simulink model "Plant_sim"  (R2022b)
settings: Solver=VariableStepAuto  StartTime=0.0  StopTime=10.0  RelTol=1e-3
PreLoadFcn:
  | param
values from neighbouring files (symbols this model uses):
  b = 0.1    [init_cond.m]    (also in param.m)
  Ce = 1.2    [init_cond.m]    (also in param.m)
  Cm = 1.2    [init_cond.m]    (also in param.m)
  J = 0.04    [init_cond.m]    (also in param.m)
  Le = 0.01    [init_cond.m]    (also in param.m)
  Lf = 0.01    [init_cond.m]    (also in param.m)
  Lrot = Le+Lf    (= 0.02)    [init_cond.m]    (also in param.m)
  Re = 4    [init_cond.m]    (also in param.m)
  Rf = 0.9    [init_cond.m]    (also in param.m)
  Rrot = Re+Rf    (= 4.9)    [init_cond.m]    (also in param.m)
libraries: fl_lib x5, nesl_utility x4, ee_lib x1
settings Model: Creator=antsupove  LastModifiedBy=antsupove
settings DebuggingCC: UnconnectedInputMsg=warning  UnconnectedOutputMsg=warning  UnconnectedLineMsg=warning
settings ModelReferenceCC: EnableRefExpFcnMdlSchedulingChecks=on
settings RTWCC: DLArmComputeVersion=19.05

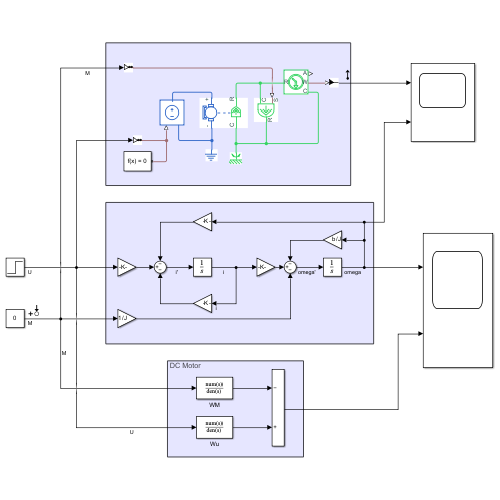
[thumbnail: Simulink's stored preview of the top-level diagram]
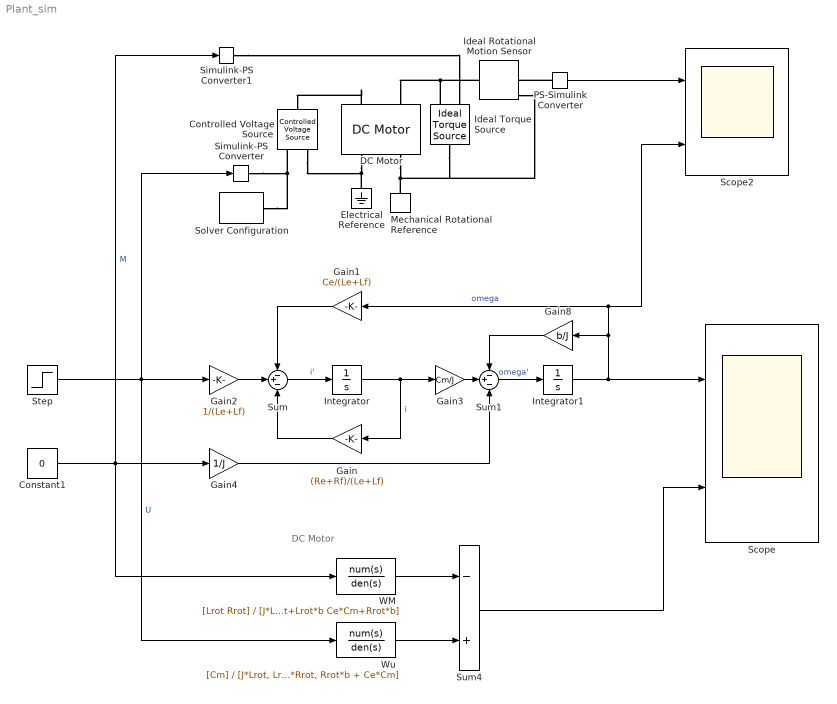
== system Plant_sim ==
  note: DC Motor
  Constant1 : Constant  Value=0
  Controlled Voltage Source : fl_lib/Electrical/Electrical Sources/Controlled Voltage Source
  DC Motor : ee_lib/Electromechanical/Brushed Motors/DC Motor  field_option=ee.enum.field_option.pm  Rf=100 Ohm  Lf=1 H  Laf=0.15 H  If0=0 A  parameterization=ee.enum.dcparam_option.circuit_param  Ra=Rrot Ohm  La=Lrot H  emf_or_torque=ee.enum.emf_or_torque.ki  Kv=0.072e-3 V/rpm  Ki=Cm N*m/A  T_stall=0.24e-3 N*m  w_max=19100 rpm  w_rated=15000 rpm  P_rated=0.08 W  V_rated=1.5 V  lam_param=ee.enum.lam_param.damping  i_noload=0 A  V_i_noload=1.5 V  J=J kg*m^2  lam=b N*m/(rad/s)  speed0=0 rad/s  enable_fault_armature=simscape.enum.onoff.off  rev_faulted=1 / 3  G_faulted_armature=1e-5 S  fault_trigger_armature=ee.enum.faults.faultTrigger.temporal  t_fault_armature=1 s  max_permissible_current_armature=inf A  t_fail_on_current_armature=1 s  enable_fault_field=simscape.enum.onoff.off  G_faulted_field=1e-5 S  fault_trigger_field=ee.enum.faults.faultTrigger.temporal  t_fault_field=1 s  max_permissible_current_field=inf A  t_fail_on_current_field=1 s  fault_action=simscape.enum.assert.action.none  alpha=3.93e-3 1/K  Tmeas=25 degC  thermal_mass=100 J/K  initial_temperature=25 degC
  Electrical Reference : fl_lib/Electrical/Electrical Elements/Electrical Reference
  Gain : Gain  Gain=(Re+Rf)/(Le+Lf)
  Gain1 : Gain  Gain=Ce/(Le+Lf)
  Gain2 : Gain  Gain=1/(Le+Lf)
  Gain3 : Gain  Gain=Cm/J
  Gain4 : Gain  Gain=1/J
  Gain8 : Gain  Gain=b/J
  Ideal Rotational Motion Sensor : fl_lib/Mechanical/Mechanical Sensors/Ideal Rotational Motion Sensor  reference=foundation.enum.MeasurementReference.difference  acceleration_port=false  velocity_port=true  position_port=true  wrap_angle=simscape.enum.onoff.off  offset=0 rad
  Ideal Torque Source : fl_lib/Mechanical/Mechanical Sources/Ideal Torque Source
  Integrator : Integrator
  Integrator1 : Integrator
  Mechanical Rotational Reference : fl_lib/Mechanical/Rotational Elements/Mechanical Rotational Reference
  PS-Simulink Converter : nesl_utility/PS-Simulink Converter  PhysicalDomain=network_engine_domain  SubClassName=ps_output  LeftPortType=input  RightPortType=output  PseudoPeriodic=off  Frequencies=[]  VectorFormat=1-D array  Unit=inherit  AffineConversion=off
  Scope : Scope  NumInputPorts=2
  Scope2 : Scope  NumInputPorts=2
  Simulink-PS Converter : nesl_utility/Simulink-PS Converter  PhysicalDomain=network_engine_domain  SubClassName=ps_input  LeftPortType=input  RightPortType=output  PseudoPeriodic=off  Frequencies=[]  NoiseDistribution=none  NoiseParameters=[]  Unit=1  AffineConversion=off  FilteringAndDerivatives=filter  SimscapeFilterOrder=2  InputFilterTimeConstant=0.001  UdotUserProvided=0
  Simulink-PS Converter1 : nesl_utility/Simulink-PS Converter  PhysicalDomain=network_engine_domain  SubClassName=ps_input  LeftPortType=input  RightPortType=output  PseudoPeriodic=off  Frequencies=[]  NoiseDistribution=none  NoiseParameters=[]  Unit=1  AffineConversion=off  FilteringAndDerivatives=filter  SimscapeFilterOrder=2  InputFilterTimeConstant=0.001  UdotUserProvided=0
  Solver Configuration : nesl_utility/Solver Configuration  PhysicalDomain=network_engine_domain  SubClassName=solver  LeftPortType=input  RightPortType=generic  Tones=[]  Harmonics=[]  SimulateNoise=off  Profile=off  UseLocalSampling=off  EnableSwitchedLinearOptims=on  FrequencyDomain=off  UseCCode=off  RelTol=0.001  AbsTol=1e-06  MinStep=1e-09  ToWorkspace=off  RevertToSquareIcSolve=off  NumHomotopyIterations=100  PhasorMode=off  PhasorModeNumHarmonics=1  ConsistencySolver=NEWTON_FTOL  IndexReductionMethod=DerivativeReplacement  DoDC=off  ResidualTolerance=1e-09  ConsistencyTolSource=GLOBAL  ConsistencyAbsTol=0.001  ConsistencyRelTol=0.001  ConsistencyTolFactor=0.001  UseLocalSolver=off  LocalSolverChoice=NE_BACKWARD_EULER_ADVANCER  ResolveIndetEquations=on  FunctionEvalNumThread=1  LocalSolverSampleTime=0.001  DoFixedCost=off  MaxNonlinIter=3  MaxModeIter=2  ComputeImpulses=off  ImpulseIterations=2  LinearAlgebra=auto  LinearAlgebraNumThread=0  EquationFormulation=NE_TIME_EF  DelaysMemoryBudget=1024  AutomaticFiltering=on  FilteringTimeConstant=0.001  PartitionStorageMethod=AS_NEEDED  PartitionMemoryBudget=1024  PartitionMethod=ROBUST
  Step : Step  SampleTime=0
  Sum : Sum  Inputs=-+-
  Sum1 : Sum  Inputs=-+-
  Sum4 : Sum  Inputs=-+
  WM : TransferFcn  Numerator=[Lrot Rrot]  Denominator=[J*Lrot J*Rrot+Lrot*b Ce*Cm+Rrot*b]
  Wu : TransferFcn  Numerator=[Cm]  Denominator=[J*Lrot, Lrot*b + J*Rrot, Rrot*b + Ce*Cm]
  wires:
  Sum/1 -> Integrator/1  "i'"
  Integrator/1 -> Gain/1, Gain3/1  "i"
  Integrator1/1 -> Scope2/2, Gain1/1, Gain8/1, Scope/1  "omega"
  Gain/1 -> Sum/3
  Gain1/1 -> Sum/1
  Gain2/1 -> Sum/2
  Sum1/1 -> Integrator1/1  "omega'"
  Step/1 -> Simulink-PS Converter/1, Gain2/1, Wu/1  "U"
  Sum4/1 -> Scope/2
  WM/1 -> Sum4/1
  Wu/1 -> Sum4/2
  PS-Simulink Converter/1 -> Scope2/1
  Constant1/1 -> WM/1, Gain4/1, Simulink-PS Converter1/1  "M"
  Gain3/1 -> Sum1/2
  Gain8/1 -> Sum1/1
  Gain4/1 -> Sum1/3
  connections:
  DC Motor/LConn1 -- Controlled Voltage Source/LConn1
  Electrical Reference/LConn1 -- DC Motor/RConn1 -- Controlled Voltage Source/RConn2
  Mechanical Rotational Reference/LConn1 -- Ideal Torque Source/LConn1 -- Ideal Rotational Motion Sensor/RConn1 -- DC Motor/RConn2
  Simulink-PS Converter/RConn1 -- Solver Configuration/RConn1 -- Controlled Voltage Source/RConn1
  PS-Simulink Converter/LConn1 -- Ideal Rotational Motion Sensor/RConn2
  Ideal Torque Source/RConn2 -- Ideal Rotational Motion Sensor/LConn1 -- DC Motor/LConn2
  Simulink-PS Converter1/RConn1 -- Ideal Torque Source/RConn1
